simulink model "TCS1"  (R2023a)
settings: Solver=VariableStepAuto  StartTime=0.0  StopTime=10  RelTol=1e-6
settings Model: Creator=ibaad  LastModifiedBy=ibaad
settings DebuggingCC: AlgebraicLoopMsg=none

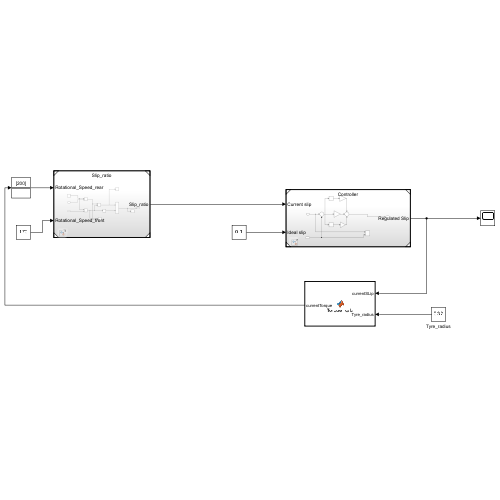
[thumbnail: Simulink's stored preview of the top-level diagram]
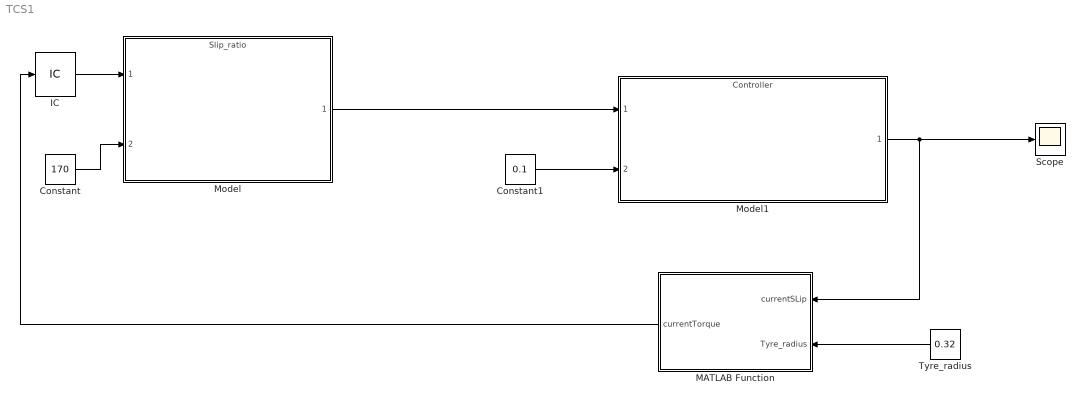
== system TCS1 ==
  Constant : Constant  Value=170
  Constant1 : Constant  Value=0.1
  IC : InitialCondition  Value=200
  MATLAB Function : MATLAB Function  TreatAsAtomicUnit=on
  Model : ModelReference  ModelNameDialog=Slip_ratio.slx  SimulationMode=Normal  ModelReferenceVersion=1.5
  Model1 : ModelReference  ModelNameDialog=Controller  SimulationMode=Normal  ModelReferenceVersion=1.8
  Scope : Scope
  Tyre_radius : Constant  Value=0.32
  wires:
  Model1/1 -> MATLAB Function/1(currentSLip), Scope/1
  Tyre_radius/1 -> MATLAB Function/2(Tyre_radius)
  MATLAB Function/1(currentTorque) -> IC/1
  Constant/1 -> Model/2
  IC/1 -> Model/1
  Model/1 -> Model1/1
  Constant1/1 -> Model1/2

== matlab function TCS1/MATLAB Function ==
  data: currentTorque output; currentSLip input; Tyre_radius input
function currentTorque = Torque_calc(currentSLip, Tyre_radius)
    % TCS_ACTIVE Summary of this function goes here

    e = exp(1); % Mathematical constant e
    % Friction curve as a function of slip ratio
    c1 = 1.2801; % Coef for dry asphalt
    c2 = 23.99; % Coef for dry asphalt
    c3 = 0.52; % Coef for dry asphalt
    Fn = 1350; % Normal force on one tire
    

 %   plot(slip_ratios, fricCoef); % Plot the entire array
 %   xlabel("Slip Ratio");
 %   ylabel("Longitudinal Friction Coefficient");
 %   title("Friction Coefficient vs. Slip Ratio Curve");
 %   grid on;% Optionally, turn the grid on for better readability


    fricCoef = c1 * (1 - exp(-c2 * currentSLip)) - c3 * currentSLip;
    currentTorque = ((fricCoef * Fn) * Tyre_radius);
end
